simulink model "Microcontroller"  (R2022b)
settings: Solver=ode1be  StartTime=0.0  StopTime=10.0  FixedStep=0.001  RelTol=1e-3
undefined symbols (not defined in the file): Kku
settings Model: Creator=Maxim Kozlov  LastModifiedBy=Maxim Kozlov
settings OptimizationCC: ReuseModelBlockBuffer=on

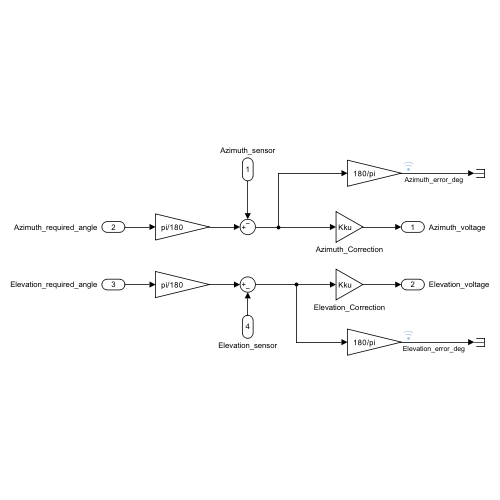
[thumbnail: Simulink's stored preview of the top-level diagram]
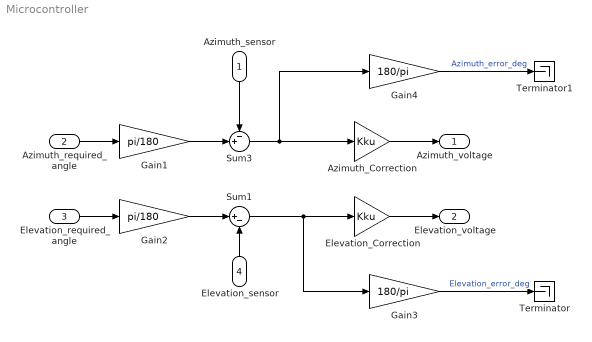
== system Microcontroller ==
  Azimuth_sensor : Inport
  Azimuth_required_angle : Inport  Port=2
  Elevation_required_angle : Inport  Port=3
  Elevation_sensor : Inport  Port=4
  Azimuth_Correction : Gain  Gain=Kku
  Elevation_Correction : Gain  Gain=Kku
  Gain1 : Gain  Gain=pi/180
  Gain2 : Gain  Gain=pi/180
  Gain3 : Gain  Gain=180/pi
  Gain4 : Gain  Gain=180/pi
  Sum1 : Sum  Inputs=|+-
  Sum3 : Sum  Inputs=-+|
  Terminator : Terminator
  Terminator1 : Terminator
  Azimuth_voltage : Outport
  Elevation_voltage : Outport  Port=2
  wires:
  Sum1/1 -> Gain3/1, Elevation_Correction/1
  Gain2/1 -> Sum1/1
  Azimuth_sensor/1 -> Sum3/1
  Elevation_sensor/1 -> Sum1/2
  Gain1/1 -> Sum3/2
  Azimuth_required_angle/1 -> Gain1/1
  Elevation_required_angle/1 -> Gain2/1
  Elevation_Correction/1 -> Elevation_voltage/1
  Azimuth_Correction/1 -> Azimuth_voltage/1
  Sum3/1 -> Gain4/1, Azimuth_Correction/1
  Gain3/1 -> Terminator/1  "Elevation_error_deg"
  Gain4/1 -> Terminator1/1  "Azimuth_error_deg"
